simulink model "Modelowanie_zawieszenia_kola"  (R2022b)
settings: Solver=VariableStepAuto  StartTime=0.0  StopTime=9  FixedStep=0.1  RelTol=1e-3
values from neighbouring files (symbols this model uses):
  A = [0 0 1 0; 0 0 0 1; -(k1+k2)/m1 k2/m1 -(c1+c2)/m1 c2/m1; k2/m2 -k2/m2 c2/m2 -c2/m2]    [Modelowanie_zawieszenie_kola.m]
  B = [c1/m1; 0; k1/m1-(c1+c2)*c1/m1^2; (c1*c2)/(m1*m2)]    [Modelowanie_zawieszenie_kola.m]
  C = diag([1 1 1 1])    [Modelowanie_zawieszenie_kola.m]
  c1 = 100    [Modelowanie_zawieszenie_kola.m]
  c2 = 2000    [Modelowanie_zawieszenie_kola.m]
  D = zeros(4, 1)    [Modelowanie_zawieszenie_kola.m]
  k1 = 370000    [Modelowanie_zawieszenie_kola.m]
  k2 = 35000    [Modelowanie_zawieszenie_kola.m]
  m1 = 90    [Modelowanie_zawieszenie_kola.m]
  m2 = 600    [Modelowanie_zawieszenie_kola.m]
settings Model: Creator=student  LastModifiedBy=Jakub
settings DebuggingCC: UnconnectedInputMsg=warning  UnconnectedOutputMsg=warning  UnconnectedLineMsg=warning
settings ModelReferenceCC: EnableRefExpFcnMdlSchedulingChecks=on
settings RTWCC: DLArmComputeVersion=19.05

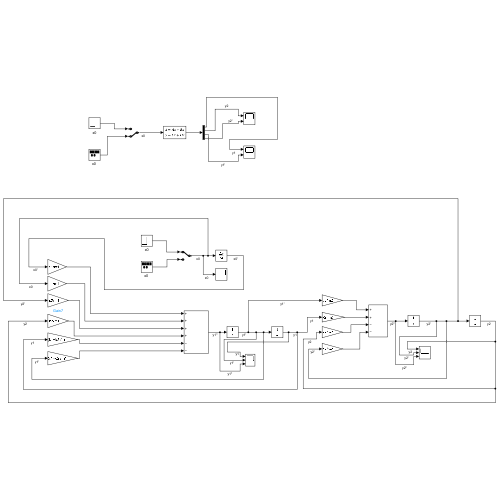
[thumbnail: Simulink's stored preview of the top-level diagram]
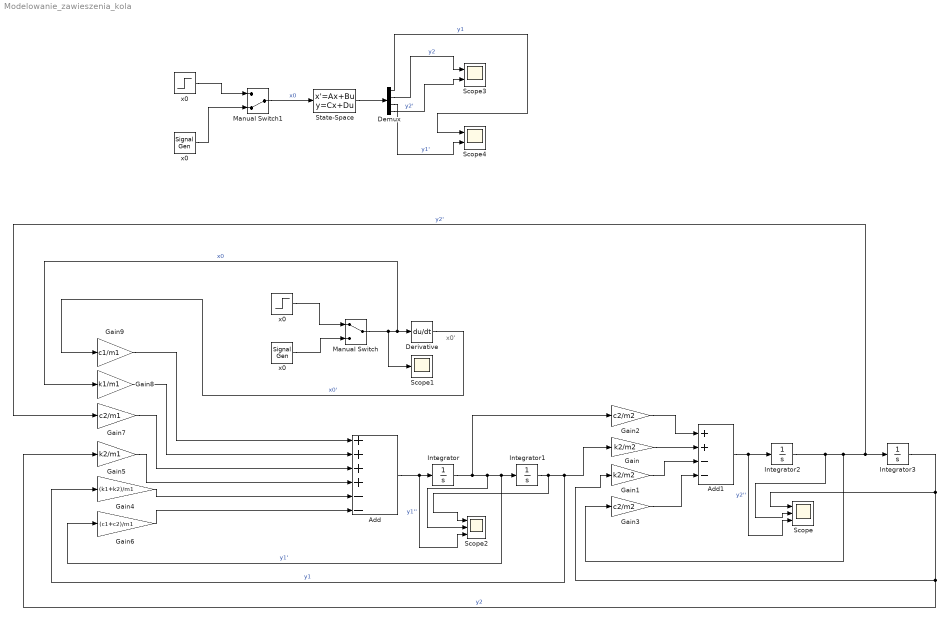
== system Modelowanie_zawieszenia_kola ==
  note: x0'
  " x0 " : Step  SampleTime=0
  " x0  " : SignalGenerator  WaveForm=square  Amplitude=0.1  Units=rad/sec
  Add : Sum  Inputs=++++--
  Add1 : Sum  Inputs=++--
  Demux : Demux
  Derivative : Derivative
  Gain : Gain  Gain=k2/m2
  Gain1 : Gain  Gain=k2/m2
  Gain2 : Gain  Gain=c2/m2
  Gain3 : Gain  Gain=c2/m2
  Gain4 : Gain  Gain=(k1+k2)/m1
  Gain5 : Gain  Gain=k2/m1
  Gain6 : Gain  Gain=(c1+c2)/m1
  Gain7 : Gain  Gain=c2/m1
  Gain8 : Gain  Gain=k1/m1
  Gain9 : Gain  Gain=c1/m1
  Integrator{,1..3} (4 alike) : Integrator
  Manual Switch : ManualSwitch
  Manual Switch1 : ManualSwitch  CurrentSetting=0
  Scope : Scope  NumInputPorts=3
  Scope1 : Scope
  Scope2 : Scope  NumInputPorts=3
  Scope3 : Scope  NumInputPorts=2
  Scope4 : Scope  NumInputPorts=2
  State-Space : StateSpace  A=A  B=B  C=C  D=D  InitialCondition=0  ParameterTunability=Optimized
  x0 : Step  SampleTime=0
  "x0 " : SignalGenerator  WaveForm=square  Amplitude=0.1  Units=rad/sec
  wires:
  Add/1 -> Scope2/3, Integrator/1  "y1''"
  Integrator/1 -> Gain2/1, Scope2/2, Gain6/1, Integrator1/1  "y1'"
  Integrator1/1 -> Gain/1, Gain4/1, Scope2/1  "y1"
  Add1/1 -> Integrator2/1, Scope/3  "y2''"
  Integrator2/1 -> Integrator3/1, Gain7/1, Gain3/1, Scope/2  "y2'"
  Integrator3/1 -> Gain1/1, Gain5/1, Scope/1  "y2"
  Gain/1 -> Add1/2
  Gain1/1 -> Add1/3
  Gain2/1 -> Add1/1
  Gain3/1 -> Add1/4
  Gain4/1 -> Add/5
  Gain6/1 -> Add/6
  Gain5/1 -> Add/4
  Gain7/1 -> Add/3
  x0/1 -> Manual Switch/1
  "x0 "/1 -> Manual Switch/2
  Manual Switch/1 -> Scope1/1, Derivative/1, Gain8/1  "x0"
  Derivative/1 -> Gain9/1  "x0'"
  Gain8/1 -> Add/2
  Gain9/1 -> Add/1
  " x0  "/1 -> Manual Switch1/2
  " x0 "/1 -> Manual Switch1/1
  Manual Switch1/1 -> State-Space/1  "x0"
  State-Space/1 -> Demux/1
  Demux/1 -> Scope4/1  "y1"
  Demux/2 -> Scope3/1  "y2"
  Demux/3 -> Scope4/2  "y1'"
  Demux/4 -> Scope3/2  "y2'"
